simulink model "DescritMotorModels"  (R2016b)
settings: Solver=FixedStepAuto  StartTime=0.0  StopTime=11.96  FixedStep=0.0001  RelTol=1e-3  EnableMultiTasking=on
undefined symbols (not defined in the file): CAL_B_NmPerW, CAL_flux_e, CAL_flux_t, CAL_Inertia_J, CAL_Re_ohm, CAL_SAMPLE_TIME, CAL_SimInduct_H, sigbuilder_block, Z0, Z1, Z2, Znom
libraries: simulink x4
settings Model: Creator=oelkawok  LastModifiedBy=oelkawok
settings DataIOCC: SaveFormat=StructureWithTime
settings OptimizationCC: DefaultParameterBehavior=Inlined  LifeSpan=1
settings DebuggingCC: SFUnexpectedBacktrackingDiag=warning  SFNoUnconditionalDefaultTransitionDiag=warning  SFExecutionAtInitializationDiag=none
settings HardwareCC: ProdLongLongMode=on
settings RTWCC: SystemTargetFile=ert.tlc  TemplateMakefile=ert_default_tmf  Description=Embedded Coder  GenerateReport=on  IncludeHyperlinkInReport=on  LaunchReport=on  GenerateTraceInfo=on  GenerateTraceReport=on  GenerateTraceReportSl=on  GenerateTraceReportSf=on  GenerateTraceReportEml=on
settings CodeAppCC: ForceParamTrailComments=on  IgnoreCustomStorageClasses=off  OperatorAnnotations=on  SimulinkDataObjDesc=on  SFDataObjDesc=on  MATLABFcnDesc=on  InsertBlockDesc=on  MATLABSourceComments=on
settings ERTTargetCC: GenerateSampleERTMain=on  InlinedParameterPlacement=NonHierarchical  ERTCustomFileTemplate=example_file_process.tlc
settings ConfigComp: CovMetricSettings=dw  CovHtmlReporting=on  CovSaveCumulativeToWorkspaceVar=on  CovSaveSingleToWorkspaceVar=on  CovExternalEMLEnable=off

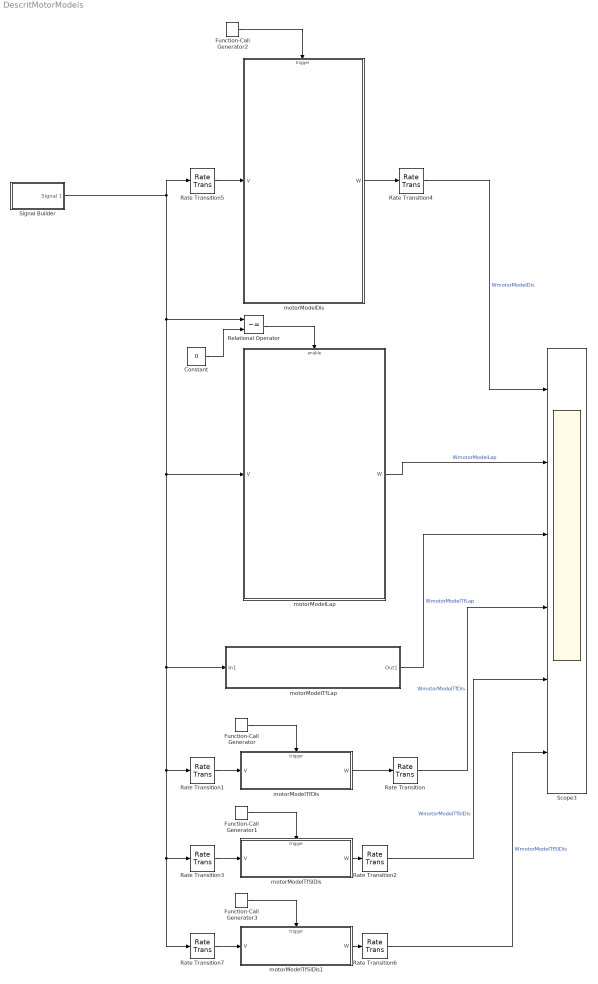
== system DescritMotorModels ==
  Constant : Constant  Value=0
  Function-Call Generator{,1..3} (4 alike) : simulink/Ports & Subsystems/Function-Call Generator  sample_time=CAL_SAMPLE_TIME  numberOfIterations=1
  Rate Transition{,1..7} (8 alike) : RateTransition
  Relational Operator : RelationalOperator  Operator=~=  OutDataTypeStr=boolean  RndMeth=Simplest
  Scope3 : Scope  NumInputPorts=6
  Signal Builder : Subsystem  Tag=STV Subsys  LoadFcn=sigbuilder_block('load',[437.4 186 550.8 400.2 ]);  StartFcn=sigbuilder_block('start');  StopFcn=sigbuilder_block('stop');  ClipboardFcn=sigbuilder_block('clipboard');  mask(Sigbuilder block){tuvar=[0:10]}
      mask help: Simulink:masks:SigbuilderBlock_MD
      mask init:
      | if ~strcmp(get_param(bdroot(gcbh),'SimulationStatus'),'stopped') tuvar = sigbuilder_block('maskInit'); end
      settings: CopyFcn=sigbuilder_block('copy');  DeleteFcn=sigbuilder_block('delete');  ModelCloseFcn=sigbuilder_block('modelClose');  PreSaveFcn=sigbuilder_block('preSave');  PauseFcn=sigbuilder_block('pause');  ContinueFcn=sigbuilder_block('continue');  NameChangeFcn=sigbuilder_block('namechange');  OpenFcn=sigbuilder_block('open',[437.4 186 550.8 400.2 ]);  CloseFcn=sigbuilder_block('close');
      mask Display: plot(0, 0, 100, 100,[2, 2, 32, 32, 2], [68, 8, 8, 68, 68],[32, 2], [38, 38], [32, 19, 2],[53, 60, 44], [32, 17, 17, 2],[16, 16, 31, 31]);txt = getActiveGroup(gcbh);text(2, 100, txt,'verticalAlignment', 'top');
  motorModelDis : Subsystem
  motorModelLap : Subsystem
  motorModelTfDis : Subsystem
  motorModelTfLap : Subsystem
  motorModelTfSlDis : Subsystem
  motorModelTfSlDis1 : Subsystem
  wires:
  Signal Builder/1(Signal 1) -> motorModelTfLap/1(In1), Rate Transition7/1, Rate Transition3/1, Rate Transition1/1, motorModelLap/1(V), Relational Operator/1, Rate Transition5/1
  motorModelTfDis/1(W) -> Rate Transition/1
  Function-Call Generator/1 -> motorModelTfDis/Trigger
  Rate Transition1/1 -> motorModelTfDis/1(V)
  motorModelTfSlDis/1(W) -> Rate Transition2/1
  Function-Call Generator1/1 -> motorModelTfSlDis/Trigger
  Rate Transition3/1 -> motorModelTfSlDis/1(V)
  Rate Transition/1 -> Scope3/4  "WmotorModelTfDis"
  Rate Transition2/1 -> Scope3/5  "WmotorModelTfSlDis"
  motorModelTfLap/1(Out1) -> Scope3/3  "WmotorModelTfLap"
  motorModelDis/1(W) -> Rate Transition4/1
  Constant/1 -> Relational Operator/2
  Relational Operator/1 -> motorModelLap/Enable
  Function-Call Generator2/1 -> motorModelDis/Trigger
  Rate Transition4/1 -> Scope3/1  "WmotorModelDis"
  Rate Transition5/1 -> motorModelDis/1(V)
  motorModelTfSlDis1/1(W) -> Rate Transition6/1
  Function-Call Generator3/1 -> motorModelTfSlDis1/Trigger
  Rate Transition7/1 -> motorModelTfSlDis1/1(V)
  Rate Transition6/1 -> Scope3/6  "WmotorModelTfSlDis"
  motorModelLap/1(W) -> Scope3/2  "WmotorModelLap"

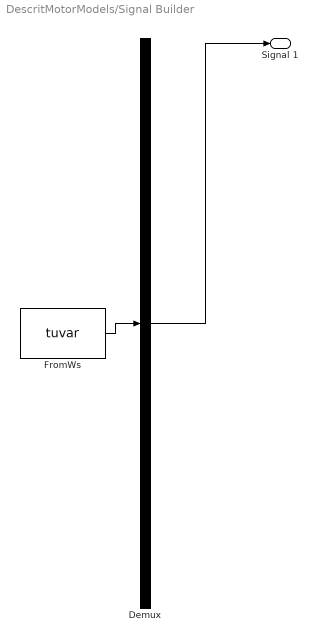
== system DescritMotorModels/Signal Builder ==
  Demux : Demux  Tag=STV Demux  Outputs=1
  FromWs : FromWorkspace  Tag=STV FromWs  VariableName=tuvar  SampleTime=0
      SigBuilderData=|
      | common.afterFinalStr = 'Extrapolate'
      | common.sampleTime = 0
      | dataSet.timeRange = [0 11.96]
      | dataSet.name = 'Group 1'
      | sbobj.Groups.Name = 'Group 1'
      | sbobj.Groups.Signals.Name = 'Signal 1'
      | sbobj.Groups.Signals.XData = [0 3 3 6 6 9 9 11.96]
      | sbobj.Groups.Signals.YData = [7.058823529 7.058823529 -7.058823529 -7.058823529 2.352941176 2.352941176 -2.352941176 -2.352941176]
      | sbobj.Groups.TimeRange = [0 11.96]
  Signal 1 : Outport  Tag=STV Outport
  wires:
  Demux/1 -> Signal 1/1
  FromWs/1 -> Demux/1

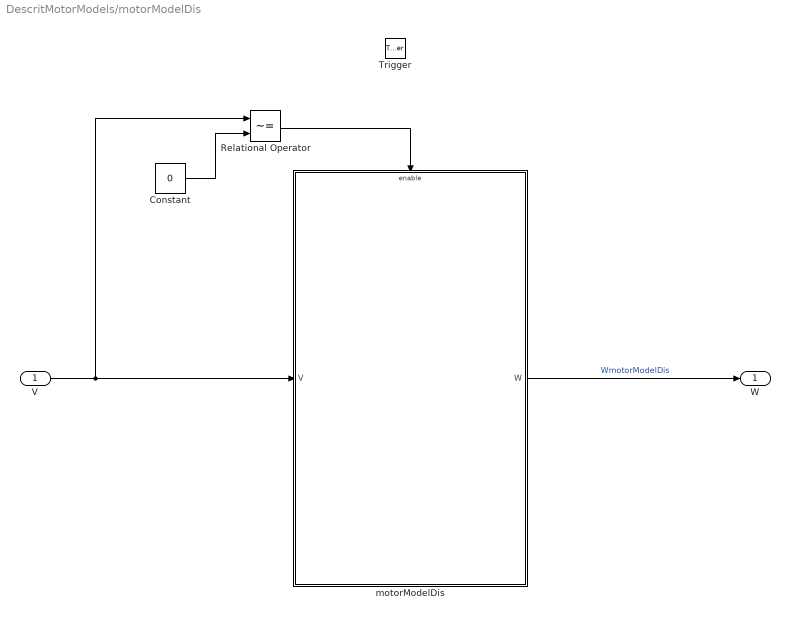
== system DescritMotorModels/motorModelDis ==
  V : Inport
  Trigger : TriggerPort  TriggerType=function-call  VariantControl=Variant  PortDimensions=1
  Constant : Constant  Value=0
  Relational Operator : RelationalOperator  Operator=~=  OutDataTypeStr=boolean  RndMeth=Simplest
  motorModelDis : Subsystem
  W : Outport
  wires:
  Relational Operator/1 -> motorModelDis/Enable
  Constant/1 -> Relational Operator/2
  motorModelDis/1(W) -> W/1  "WmotorModelDis"
  V/1 -> motorModelDis/1(V), Relational Operator/1

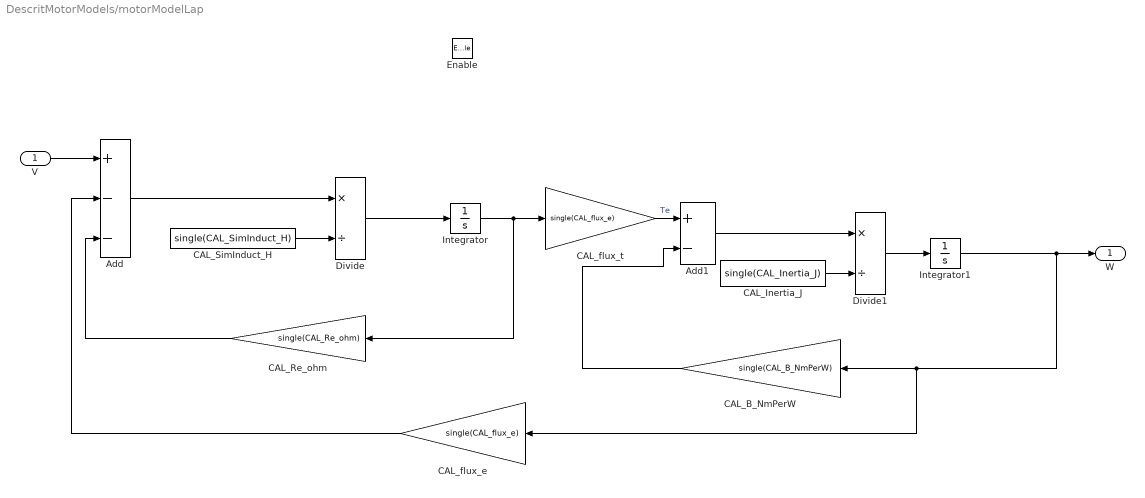
== system DescritMotorModels/motorModelLap ==
  V : Inport
  Enable : EnablePort  StatesWhenEnabling=reset
  Add : Sum  Inputs=+--
  Add1 : Sum  Inputs=+-
  CAL_B_NmPerW : Gain  Gain=single(CAL_B_NmPerW)
  CAL_Inertia_J : Constant  Value=single(CAL_Inertia_J)
  CAL_Re_ohm : Gain  Gain=single(CAL_Re_ohm)
  CAL_SimInduct_H : Constant  Value=single(CAL_SimInduct_H)
  CAL_flux_e : Gain  Gain=single(CAL_flux_e)
  CAL_flux_t : Gain  Gain=single(CAL_flux_e)
  Divide : Product  Inputs=*/
  Divide1 : Product  Inputs=*/
  Integrator : Integrator
  Integrator1 : Integrator
  W : Outport  OutputWhenDisabled=reset  InitialOutput=0
  wires:
  Integrator/1 -> CAL_Re_ohm/1, CAL_flux_t/1
  V/1 -> Add/1
  Integrator1/1 -> CAL_B_NmPerW/1, CAL_flux_e/1, W/1
  CAL_Re_ohm/1 -> Add/3
  Divide1/1 -> Integrator1/1
  CAL_SimInduct_H/1 -> Divide/2
  CAL_Inertia_J/1 -> Divide1/2
  CAL_flux_t/1 -> Add1/1  "Te"
  CAL_flux_e/1 -> Add/2
  Add1/1 -> Divide1/1
  CAL_B_NmPerW/1 -> Add1/2
  Divide/1 -> Integrator/1
  Add/1 -> Divide/1

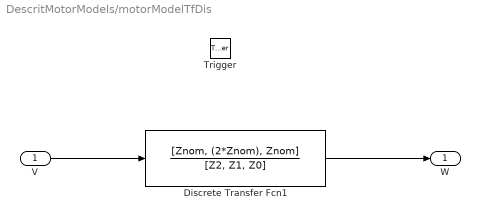
== system DescritMotorModels/motorModelTfDis ==
  V : Inport
  Trigger : TriggerPort  TriggerType=function-call  VariantControl=Variant  PortDimensions=1
  Discrete Transfer Fcn1 : DiscreteTransferFcn  Numerator=[Znom, (2*Znom), Znom]  Denominator=[Z2, Z1, Z0]
  W : Outport
  wires:
  Discrete Transfer Fcn1/1 -> W/1
  V/1 -> Discrete Transfer Fcn1/1

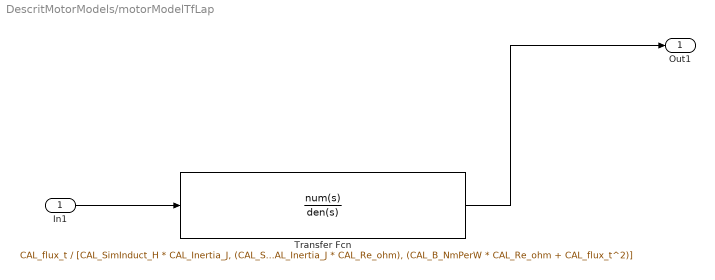
== system DescritMotorModels/motorModelTfLap ==
  In1 : Inport
  Transfer Fcn : TransferFcn  Numerator=CAL_flux_t  Denominator=[CAL_SimInduct_H * CAL_Inertia_J, (CAL_SimInduct_H * CAL_B_NmPerW + CAL_Inertia_J * CAL_Re_ohm), (CAL_B_NmPerW * CAL_Re_ohm + CAL_flux_t^2)]
  Out1 : Outport
  wires:
  In1/1 -> Transfer Fcn/1
  Transfer Fcn/1 -> Out1/1

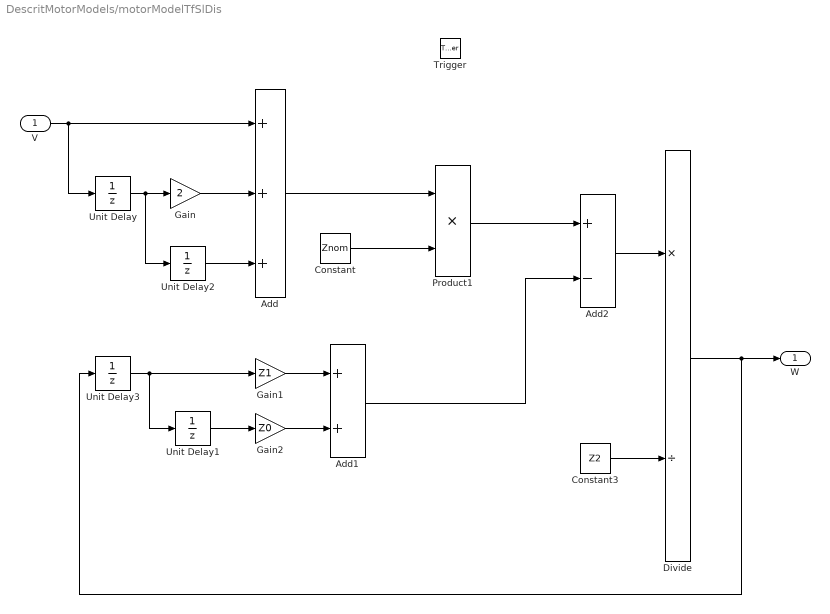
== system DescritMotorModels/motorModelTfSlDis ==
  V : Inport
  Trigger : TriggerPort  TriggerType=function-call  VariantControl=Variant  PortDimensions=1
  Add : Sum  Inputs=+++
  Add1 : Sum
  Add2 : Sum  Inputs=+-
  Constant : Constant  Value=Znom
  Constant3 : Constant  Value=Z2
  Divide : Product  Inputs=*/
  Gain : Gain  Gain=2
  Gain1 : Gain  Gain=Z1
  Gain2 : Gain  Gain=Z0
  Product1 : Product
  Unit Delay{,1..3} (4 alike) : UnitDelay  SampleTime=-1
  W : Outport
  wires:
  V/1 -> Unit Delay/1, Add/1
  Unit Delay/1 -> Unit Delay2/1, Gain/1
  Divide/1 -> W/1, Unit Delay3/1
  Constant/1 -> Product1/2
  Gain/1 -> Add/2
  Unit Delay2/1 -> Add/3
  Add/1 -> Product1/1
  Product1/1 -> Add2/1
  Unit Delay3/1 -> Unit Delay1/1, Gain1/1
  Gain1/1 -> Add1/1
  Unit Delay1/1 -> Gain2/1
  Gain2/1 -> Add1/2
  Add1/1 -> Add2/2
  Add2/1 -> Divide/1
  Constant3/1 -> Divide/2

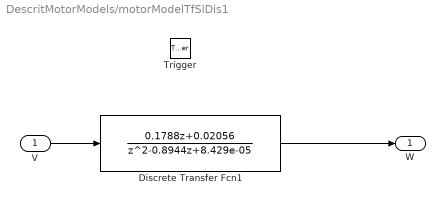
== system DescritMotorModels/motorModelTfSlDis1 ==
  V : Inport
  Trigger : TriggerPort  TriggerType=function-call  VariantControl=Variant  PortDimensions=1
  Discrete Transfer Fcn1 : DiscreteTransferFcn  Numerator=[0.1788 , 0.02056]  Denominator=[1, -0.8944, 8.429e-05]
  W : Outport
  wires:
  V/1 -> Discrete Transfer Fcn1/1
  Discrete Transfer Fcn1/1 -> W/1

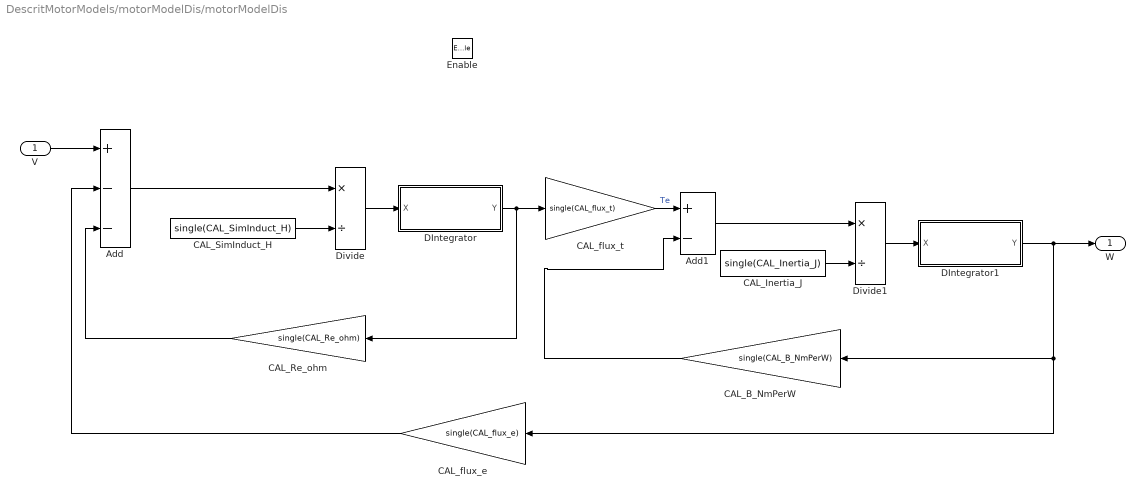
== system DescritMotorModels/motorModelDis/motorModelDis ==
  V : Inport
  Enable : EnablePort  StatesWhenEnabling=reset
  Add : Sum  Inputs=+--
  Add1 : Sum  Inputs=+-
  CAL_B_NmPerW : Gain  Gain=single(CAL_B_NmPerW)
  CAL_Inertia_J : Constant  Value=single(CAL_Inertia_J)
  CAL_Re_ohm : Gain  Gain=single(CAL_Re_ohm)
  CAL_SimInduct_H : Constant  Value=single(CAL_SimInduct_H)
  CAL_flux_e : Gain  Gain=single(CAL_flux_e)
  CAL_flux_t : Gain  Gain=single(CAL_flux_t)
  DIntegrator : Subsystem
  DIntegrator1 : Subsystem
  Divide : Product  Inputs=*/
  Divide1 : Product  Inputs=*/
  W : Outport  OutputWhenDisabled=reset  InitialOutput=0
  wires:
  Add/1 -> Divide/1
  CAL_B_NmPerW/1 -> Add1/2
  Add1/1 -> Divide1/1
  CAL_flux_e/1 -> Add/2
  CAL_flux_t/1 -> Add1/1  "Te"
  CAL_Inertia_J/1 -> Divide1/2
  CAL_SimInduct_H/1 -> Divide/2
  CAL_Re_ohm/1 -> Add/3
  V/1 -> Add/1
  Divide/1 -> DIntegrator/1(X)
  DIntegrator/1(Y) -> CAL_Re_ohm/1, CAL_flux_t/1
  Divide1/1 -> DIntegrator1/1(X)
  DIntegrator1/1(Y) -> CAL_flux_e/1, CAL_B_NmPerW/1, W/1

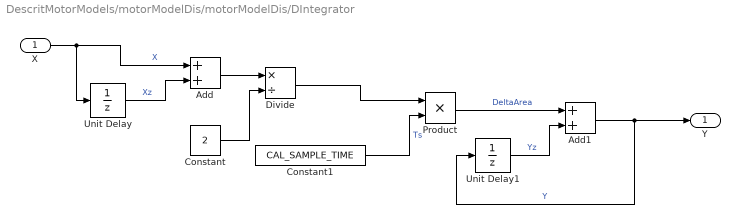
== system DescritMotorModels/motorModelDis/motorModelDis/DIntegrator ==
  X : Inport
  Add : Sum
  Add1 : Sum
  Constant : Constant  Value=2
  Constant1 : Constant  Value=CAL_SAMPLE_TIME
  Divide : Product  Inputs=*/
  Product : Product
  Unit Delay : UnitDelay  SampleTime=-1
  Unit Delay1 : UnitDelay  SampleTime=-1
  Y : Outport
  wires:
  Unit Delay/1 -> Add/2  "Xz"
  X/1 -> Unit Delay/1, Add/1  "X"
  Add/1 -> Divide/1
  Constant/1 -> Divide/2
  Constant1/1 -> Product/2  "Ts"
  Divide/1 -> Product/1
  Product/1 -> Add1/1  "DeltaArea"
  Add1/1 -> Unit Delay1/1, Y/1  "Y"
  Unit Delay1/1 -> Add1/2  "Yz"

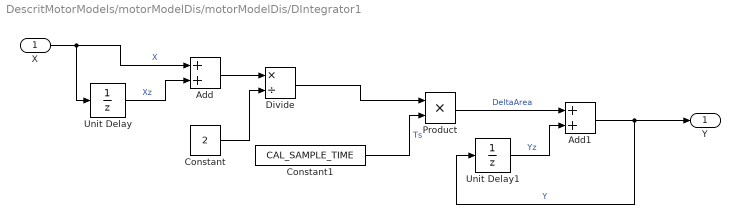
== system DescritMotorModels/motorModelDis/motorModelDis/DIntegrator1 ==
  X : Inport
  Add : Sum
  Add1 : Sum
  Constant : Constant  Value=2
  Constant1 : Constant  Value=CAL_SAMPLE_TIME
  Divide : Product  Inputs=*/
  Product : Product
  Unit Delay : UnitDelay  SampleTime=-1
  Unit Delay1 : UnitDelay  SampleTime=-1
  Y : Outport
  wires:
  Unit Delay1/1 -> Add1/2  "Yz"
  Add1/1 -> Y/1, Unit Delay1/1  "Y"
  Product/1 -> Add1/1  "DeltaArea"
  Divide/1 -> Product/1
  Constant1/1 -> Product/2  "Ts"
  Constant/1 -> Divide/2
  Add/1 -> Divide/1
  X/1 -> Add/1, Unit Delay/1  "X"
  Unit Delay/1 -> Add/2  "Xz"
